simulink model "modelo_segundaordem_fr"  (R2020a)
settings: Solver=VariableStepAuto  StartTime=0.0  StopTime=10.0  RelTol=1e-3
settings Model: Creator=luis  LastModifiedBy=luis

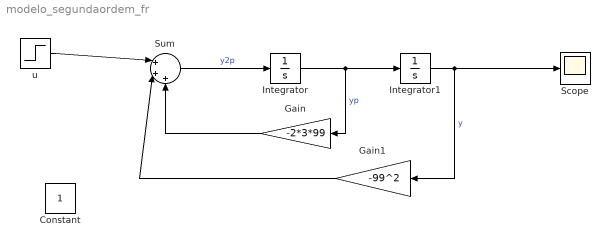
== system modelo_segundaordem_fr ==
  Constant : Constant
  Gain : Gain  Gain=-2*3*99
  Gain1 : Gain  Gain=-99^2
  Integrator : Integrator
  Integrator1 : Integrator
  Scope : Scope
  Sum : Sum  Inputs=|+++
  u : Step  Time=0.25  After=100*99^2  SampleTime=0
  wires:
  Integrator/1 -> Integrator1/1, Gain/1  "yp"
  Integrator1/1 -> Gain1/1, Scope/1  "y"
  Sum/1 -> Integrator/1  "y2p"
  u/1 -> Sum/1
  Gain/1 -> Sum/3
  Gain1/1 -> Sum/2
